simulink model "ControlSystemSimulink"  (R2024a)
settings: Solver=VariableStepAuto  StartTime=0.0  StopTime=100  RelTol=1e-3
InitFcn:
  | Ra = 1;
  | La = 0.5;
  | J = 0.01;
  | b= 0.1;
  | Kt = 0.01;
  | Kb = 0.01;
  | Ke = 0.01;
  | Kp = 6;
  | Ki = 20;
  | Kd = 0.08;
settings Model: Creator=buttrakd  LastModifiedBy=buttrakd

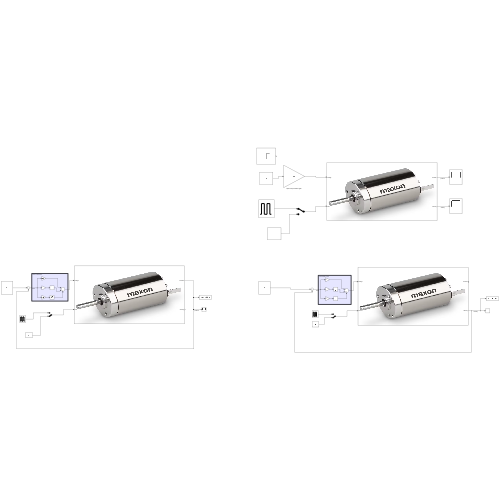
[thumbnail: Simulink's stored preview of the top-level diagram]
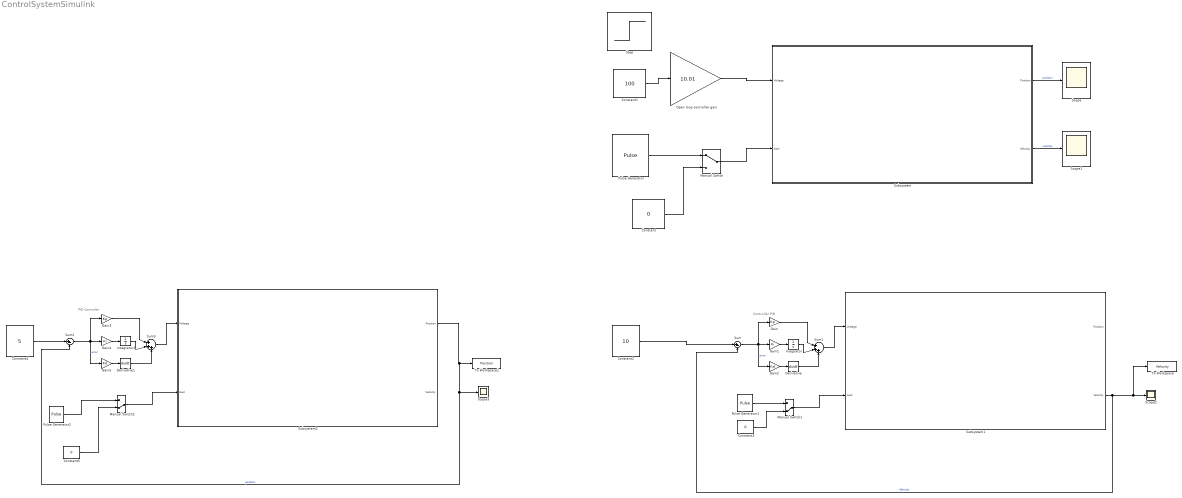
== system ControlSystemSimulink ==
  note: PID Controler
  note: Controller PID
  Constant : Constant  Value=0
  Constant1 : Constant  Value=100
  Constant2 : Constant  Value=10
  Constant3 : Constant  Value=0
  Constant4 : Constant  Value=5
  Constant5 : Constant  Value=0
  Derivative : Derivative
  Derivative1 : Derivative
  Gain : Gain  Gain=Kp
  Gain1 : Gain  Gain=Ki
  Gain2 : Gain  Gain=Kd
  Gain3 : Gain  Gain=Kp
  Gain4 : Gain  Gain=Ki
  Gain5 : Gain  Gain=Kd
  Integrator : Integrator
  Integrator1 : Integrator
  Manual Switch : ManualSwitch
  Manual Switch1 : ManualSwitch  CurrentSetting=0
  Manual Switch2 : ManualSwitch  CurrentSetting=0
  Open loop controller gain : Gain  Gain=10.01
  Pulse Generator : DiscretePulseGenerator  PulseType=Time based  Amplitude=2.5  Period=5  PulseWidth=50
  Pulse Generator1 : DiscretePulseGenerator  PulseType=Time based  Amplitude=2.5  Period=5  PulseWidth=50
  Pulse Generator2 : DiscretePulseGenerator  PulseType=Time based  Amplitude=2.5  Period=5  PulseWidth=50
  Scope{,1..3} (4 alike) : Scope
  Step : Step  SampleTime=0
  Subsystem : Subsystem
      mask Display: image('Maxon DC motor.png');
  Subsystem1 : Subsystem
      mask Display: image('Maxon DC motor.png');
  Subsystem2 : Subsystem
      mask Display: image('Maxon DC motor.png');
  Sum : Sum  Inputs=|+-
  Sum1 : Sum  Inputs=|+++
  Sum2 : Sum  Inputs=|+-
  Sum3 : Sum  Inputs=|+++
  To Workspace : ToWorkspace  VariableName=Velocity  SaveFormat=Timeseries  SampleTime=-1
  To Workspace1 : ToWorkspace  VariableName=Position  SaveFormat=Timeseries  SampleTime=-1
  wires:
  Subsystem/1(Position) -> Scope/1  "position"
  Subsystem/2(Velocity) -> Scope1/1  "velocity"
  Open loop controller gain/1 -> Subsystem/1(Voltage)
  Constant1/1 -> Open loop controller gain/1
  Pulse Generator/1 -> Manual Switch/1
  Constant/1 -> Manual Switch/2
  Manual Switch/1 -> Subsystem/2(load)
  Subsystem1/2(Velocity) -> Sum/2, To Workspace/1, Scope2/1  "Velocity"
  Constant2/1 -> Sum/1
  Sum/1 -> Gain2/1, Gain/1, Gain1/1  "error"
  Gain/1 -> Sum1/1
  Integrator/1 -> Sum1/2
  Derivative/1 -> Sum1/3
  Sum1/1 -> Subsystem1/1(Voltage)
  Manual Switch1/1 -> Subsystem1/2(load)
  Constant3/1 -> Manual Switch1/2
  Pulse Generator1/1 -> Manual Switch1/1
  Gain1/1 -> Integrator/1
  Gain2/1 -> Derivative/1
  Gain5/1 -> Derivative1/1
  Gain4/1 -> Integrator1/1
  Pulse Generator2/1 -> Manual Switch2/1
  Constant5/1 -> Manual Switch2/2
  Manual Switch2/1 -> Subsystem2/2(load)
  Sum3/1 -> Subsystem2/1(Voltage)
  Derivative1/1 -> Sum3/3
  Integrator1/1 -> Sum3/2
  Gain3/1 -> Sum3/1
  Sum2/1 -> Gain4/1, Gain3/1, Gain5/1  "error"
  Constant4/1 -> Sum2/1
  Subsystem2/1(Position) -> Sum2/2, Scope3/1, To Workspace1/1  "position"

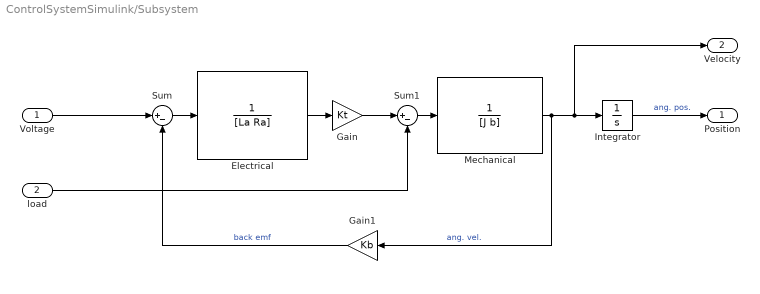
== system ControlSystemSimulink/Subsystem ==
  Voltage : Inport
  load : Inport  Port=2
  Electrical : TransferFcn  Denominator=[La Ra]
  Gain : Gain  Gain=Kt
  Gain1 : Gain  Gain=Kb
  Integrator : Integrator
  Mechanical : TransferFcn  Denominator=[J b]
  Sum : Sum  Inputs=|+-
  Sum1 : Sum  Inputs=|+-
  Position : Outport
  Velocity : Outport  Port=2
  wires:
  Mechanical/1 -> Velocity/1, Integrator/1, Gain1/1  "ang. vel."
  Gain1/1 -> Sum/2  "back emf"
  Sum1/1 -> Mechanical/1
  Gain/1 -> Sum1/1
  Sum/1 -> Electrical/1
  Electrical/1 -> Gain/1
  Voltage/1 -> Sum/1
  load/1 -> Sum1/2
  Integrator/1 -> Position/1  "ang. pos."

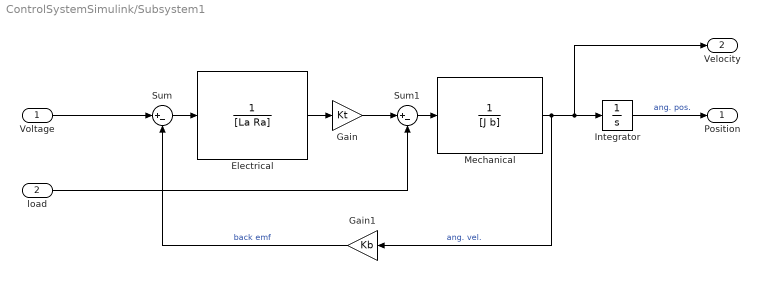
== system ControlSystemSimulink/Subsystem1 ==
  Voltage : Inport
  load : Inport  Port=2
  Electrical : TransferFcn  Denominator=[La Ra]
  Gain : Gain  Gain=Kt
  Gain1 : Gain  Gain=Kb
  Integrator : Integrator
  Mechanical : TransferFcn  Denominator=[J b]
  Sum : Sum  Inputs=|+-
  Sum1 : Sum  Inputs=|+-
  Position : Outport
  Velocity : Outport  Port=2
  wires:
  Integrator/1 -> Position/1  "ang. pos."
  load/1 -> Sum1/2
  Voltage/1 -> Sum/1
  Electrical/1 -> Gain/1
  Sum/1 -> Electrical/1
  Gain/1 -> Sum1/1
  Sum1/1 -> Mechanical/1
  Gain1/1 -> Sum/2  "back emf"
  Mechanical/1 -> Gain1/1, Integrator/1, Velocity/1  "ang. vel."

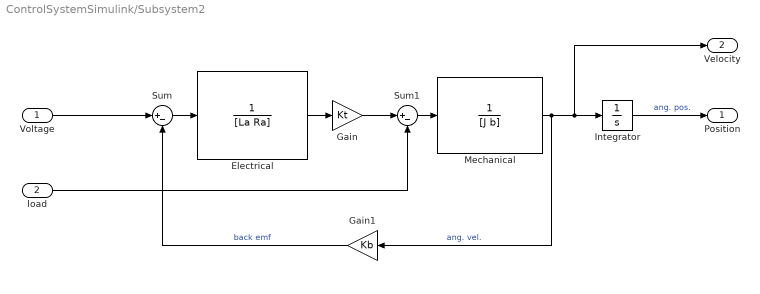
== system ControlSystemSimulink/Subsystem2 ==
  Voltage : Inport
  load : Inport  Port=2
  Electrical : TransferFcn  Denominator=[La Ra]
  Gain : Gain  Gain=Kt
  Gain1 : Gain  Gain=Kb
  Integrator : Integrator
  Mechanical : TransferFcn  Denominator=[J b]
  Sum : Sum  Inputs=|+-
  Sum1 : Sum  Inputs=|+-
  Position : Outport
  Velocity : Outport  Port=2
  wires:
  Mechanical/1 -> Velocity/1, Integrator/1, Gain1/1  "ang. vel."
  Gain1/1 -> Sum/2  "back emf"
  Sum1/1 -> Mechanical/1
  Gain/1 -> Sum1/1
  Sum/1 -> Electrical/1
  Electrical/1 -> Gain/1
  Voltage/1 -> Sum/1
  load/1 -> Sum1/2
  Integrator/1 -> Position/1  "ang. pos."
